simulink model "TotalFramework"  (Simulink 6.6)
settings: Solver=ode45  StartTime=0.0  StopTime=inf  RelTol=1e-3
libraries: xbsIndex_r4 x42, simulink x4, dspsrcs4 x1, simulink_extras x1
settings Model: Creator=student  LastModifiedBy=student

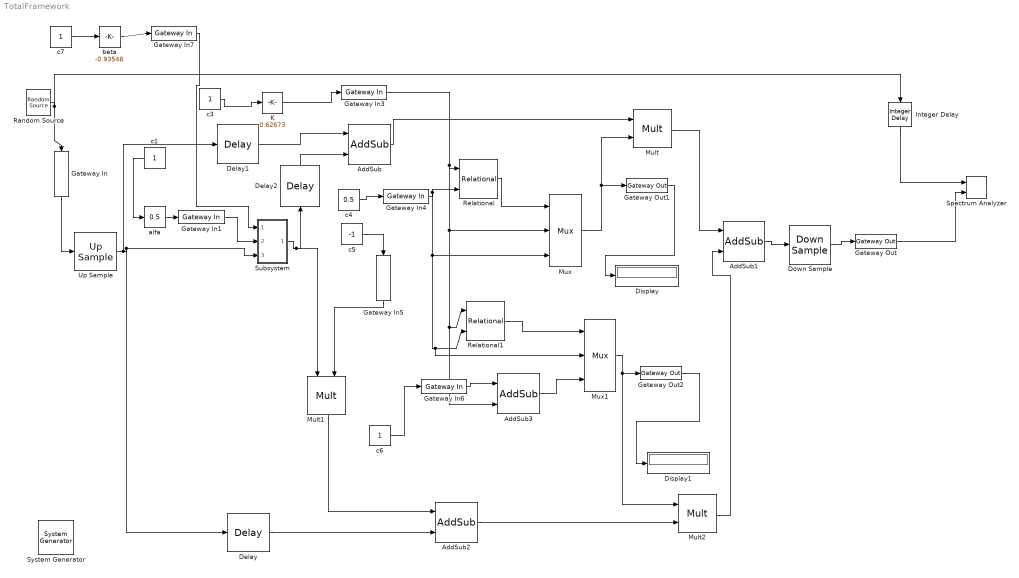
== system TotalFramework ==
  " System Generator" : xbsIndex_r4/ System Generator  Tag=genX  SystemSampleTime=-1  xilinxfamily=virtex4  part=xc4vsx35  speed=-10  package=ff668  synthesis_tool=XST  directory=./netlist  testbench=off  simulink_period=1/10  sysclk_period=10  incr_netlist=off  trim_vbits=Everywhere in SubSystem  dbl_ovrd=According to Block Masks  core_generation=According to Block Masks  run_coregen=off  deprecated_control=off  eval_field=0  block_type=sysgen
      settings: block_version=9.2.00
  AddSub : xbsIndex_r4/AddSub  mode=Addition  use_carryin=off  use_carryout=off  en=off  latency=0  precision=Full  arith_type=Unsigned  n_bits=16  bin_pt=14  quantization=Truncate  overflow=Wrap  dbl_ovrd=off  use_behavioral_HDL=off  pipelined=off  use_rpm=on  block_type=addsub
      settings: block_version=9.2.00
  AddSub1 : xbsIndex_r4/AddSub  mode=Addition  use_carryin=off  use_carryout=off  en=off  latency=2  precision=User Defined  arith_type="Signed  (2's comp)"  n_bits=16  bin_pt=14  quantization=Truncate  overflow=Wrap  dbl_ovrd=off  use_behavioral_HDL=off  pipelined=off  use_rpm=on  block_type=addsub
      settings: block_version=9.2.00
  AddSub2 : xbsIndex_r4/AddSub  mode=Addition  use_carryin=off  use_carryout=off  en=off  latency=0  precision=Full  arith_type=Unsigned  n_bits=16  bin_pt=14  quantization=Truncate  overflow=Wrap  dbl_ovrd=off  use_behavioral_HDL=off  pipelined=off  use_rpm=on  block_type=addsub
      settings: block_version=9.2.00
  AddSub3 : xbsIndex_r4/AddSub  mode=Subtraction  use_carryin=off  use_carryout=off  en=off  latency=0  precision=Full  arith_type=Unsigned  n_bits=16  bin_pt=14  quantization=Truncate  overflow=Wrap  dbl_ovrd=off  use_behavioral_HDL=off  pipelined=off  use_rpm=on  block_type=addsub
      settings: block_version=9.2.00
  Delay : xbsIndex_r4/Delay  en=off  latency=13  dbl_ovrd=off  reg_retiming=off  block_type=delay
      settings: block_version=9.2.00
  Delay1 : xbsIndex_r4/Delay  en=off  latency=13  dbl_ovrd=off  reg_retiming=off  block_type=delay
      settings: block_version=9.2.00
  Delay2 : xbsIndex_r4/Delay  Orientation=up  en=off  latency=3  dbl_ovrd=off  reg_retiming=off  block_type=delay
      settings: block_version=9.2.00
  Display : Display
  Display1 : Display
  Down Sample : xbsIndex_r4/Down Sample  sample_ratio=10  sample_phase=First Value of Frame  en=off  latency=0  dbl_ovrd=off  block_type=dsamp
      settings: block_version=9.2.00
  Gateway In : xbsIndex_r4/Gateway In  Orientation=down  arith_type="Signed  (2's comp)"  n_bits=16  bin_pt=14  quantization="Round  (unbiased: +/- Inf)"  overflow=Saturate  period=1  dbl_ovrd=off  timing_constraint=None  locs_specified=off  LOCs={}  block_type=gatewayin
      settings: infoedit="Gateway in block.  Converts inputs of type Simulink integer, double and fixed point to  Xilinx fixed point type.<P><P>Hardware notes:  In hardware these blocks become top level input ports."  block_version=9.2.00
  Gateway In{1,3..4,6..7} (5 alike) : xbsIndex_r4/Gateway In  arith_type="Signed  (2's comp)"  n_bits=16  bin_pt=14  quantization="Round  (unbiased: +/- Inf)"  overflow=Saturate  period=1  dbl_ovrd=off  timing_constraint=None  locs_specified=off  LOCs={}  block_type=gatewayin
      settings: infoedit="Gateway in block.  Converts inputs of type Simulink integer, double and fixed point to  Xilinx fixed point type.<P><P>Hardware notes:  In hardware these blocks become top level input ports."  block_version=9.2.00
  Gateway In5 : xbsIndex_r4/Gateway In  Orientation=down  arith_type="Signed  (2's comp)"  n_bits=16  bin_pt=14  quantization="Round  (unbiased: +/- Inf)"  overflow=Saturate  period=1  dbl_ovrd=off  timing_constraint=None  locs_specified=off  LOCs={}  block_type=gatewayin
      settings: infoedit="Gateway in block.  Converts inputs of type Simulink integer, double and fixed point to  Xilinx fixed point type.<P><P>Hardware notes:  In hardware these blocks become top level input ports."  block_version=9.2.00
  Gateway Out : xbsIndex_r4/Gateway Out  hdl_port=on  timing_constraint=None  locs_specified=off  LOCs={}  block_type=gatewayout
      settings: infoedit="Gateway out block.  Converts Xilinx fixed point inputs into ouputs of type Simulink integer, double, or fixed point.<P><P>Hardware notes:  In hardware these blocks become top level output ports or are discarded, depending on how they are configured."  block_version=9.2.00
  Gateway Out1 : xbsIndex_r4/Gateway Out  hdl_port=on  timing_constraint=None  locs_specified=off  LOCs={}  block_type=gatewayout
      settings: infoedit="Gateway out block.  Converts Xilinx fixed point inputs into ouputs of type Simulink integer, double, or fixed point.<P><P>Hardware notes:  In hardware these blocks become top level output ports or are discarded, depending on how they are configured."  block_version=9.2.00
  Gateway Out2 : xbsIndex_r4/Gateway Out  hdl_port=on  timing_constraint=None  locs_specified=off  LOCs={}  block_type=gatewayout
      settings: infoedit="Gateway out block.  Converts Xilinx fixed point inputs into ouputs of type Simulink integer, double, or fixed point.<P><P>Hardware notes:  In hardware these blocks become top level output ports or are discarded, depending on how they are configured."  block_version=9.2.00
  Integer Delay : simulink/Discrete/Integer Delay  Orientation=down  vinit=0.0  samptime=1  NumDelays=2
  K : simulink/Math Operations/Slider Gain  SystemSampleTime=-1  low=0  gain=0.62673  high=1
  Mult : xbsIndex_r4/Mult  precision=Full  arith_type="Signed  (2's comp)"  n_bits=16  bin_pt=14  quantization=Truncate  overflow=Wrap  en=off  latency=5  dbl_ovrd=off  use_behavioral_HDL=off  use_embedded=on  opt=Speed  optimum_pipeline=off  pipeline=on  use_rpm=on  placement_style=Triangular  block_type=mult
      settings: infoedit=Hardware notes: To use the internal pipeline stage of the dedicated multiplier you must select 'Pipeline for maximum performance'.  block_version=9.2.00
  Mult1 : xbsIndex_r4/Mult  Orientation=down  precision=Full  arith_type="Signed  (2's comp)"  n_bits=16  bin_pt=14  quantization=Truncate  overflow=Wrap  en=off  latency=3  dbl_ovrd=off  use_behavioral_HDL=off  use_embedded=on  opt=Speed  optimum_pipeline=off  pipeline=on  use_rpm=on  placement_style=Triangular  block_type=mult
      settings: infoedit=Hardware notes: To use the internal pipeline stage of the dedicated multiplier you must select 'Pipeline for maximum performance'.  block_version=9.2.00
  Mult2 : xbsIndex_r4/Mult  precision=Full  arith_type="Signed  (2's comp)"  n_bits=16  bin_pt=14  quantization=Truncate  overflow=Wrap  en=off  latency=5  dbl_ovrd=off  use_behavioral_HDL=off  use_embedded=on  opt=Speed  optimum_pipeline=off  pipeline=on  use_rpm=on  placement_style=Triangular  block_type=mult
      settings: infoedit=Hardware notes: To use the internal pipeline stage of the dedicated multiplier you must select 'Pipeline for maximum performance'.  block_version=9.2.00
  Mux : xbsIndex_r4/Mux  inputs=2  en=off  latency=0  precision=Full  arith_type=Unsigned  n_bits=16  bin_pt=14  quantization=Truncate  overflow=Wrap  dbl_ovrd=off  block_type=mux
      settings: block_version=9.2.00
  Mux1 : xbsIndex_r4/Mux  inputs=2  en=off  latency=0  precision=Full  arith_type=Unsigned  n_bits=16  bin_pt=14  quantization=Truncate  overflow=Wrap  dbl_ovrd=off  block_type=mux
      settings: block_version=9.2.00
  Random Source : dspsrcs4/Random Source  SrcType=Uniform  NormMethod=Ziggurat  CltLength=12  MinVal=-1  MaxVal=+1  MeanVal=0  VarVal=1  RepMode=Not repeatable  rawSeed=1  IsInherit=off  SampMode=Discrete  SampTime=1  SampFrame=1  DataType=Double  OutComplex=Real
  Relational : xbsIndex_r4/Relational  mode=a>b  en=off  latency=1  dbl_ovrd=off  block_type=relational
      settings: block_version=9.2.00
  Relational1 : xbsIndex_r4/Relational  mode=a>b  en=off  latency=1  dbl_ovrd=off  block_type=relational
      settings: block_version=9.2.00
  Spectrum Analyzer : simulink_extras/Additional Sinks/Spectrum Analyzer  SystemSampleTime=-1  npts=1024  fftpts=1024  HowOften=64  sampleT=1
  Subsystem : Subsystem
  Up Sample : xbsIndex_r4/Up Sample  sample_ratio=10  copy_samples=off  dbl_ovrd=off  block_type=usamp
      settings: infoedit="Up samples input data.  Inserted values  can be zeros or copies of the most recent input sample.<P><P>Hardware notes: No hardware is needed if inserted values are copies of the input sample; otherwise, a mux and single bit flip-flop are used."  block_version=9.2.00
  alfa : simulink/Math Operations/Slider Gain  SystemSampleTime=-1  low=0  gain=0.5  high=1
  beta : simulink/Math Operations/Slider Gain  SystemSampleTime=-1  low=-1  gain=-0.93548  high=1
  c1 : Constant  Orientation=left
  c3 : Constant
  c4 : Constant  Value=0.5
  c5 : Constant  Value=-1
  c6 : Constant
  c7 : Constant
  wires:
  Random Source/1 -> Gateway In/1, Integer Delay/1
  c1/1 -> alfa/1
  alfa/1 -> Gateway In1/1
  Gateway Out/1 -> Spectrum Analyzer/2
  Subsystem/1(Out1) -> Mult1/1, Delay2/1
  c3/1 -> K/1
  K/1 -> Gateway In3/1
  c4/1 -> Gateway In4/1
  Gateway In4/1 -> Relational/2, Mux/3, Relational1/2, Mux1/2
  Gateway In3/1 -> Relational/1, Mux/2, Relational1/1, AddSub3/2
  AddSub/1 -> Mult/1
  Mult/1 -> AddSub1/1
  c5/1 -> Gateway In5/1
  Gateway In5/1 -> Mult1/2
  Mult1/1 -> AddSub2/1
  Relational/1 -> Mux/1
  Gateway Out1/1 -> Display/1
  Mux/1 -> Mult/2, Gateway Out1/1
  Relational1/1 -> Mux1/1
  c6/1 -> Gateway In6/1
  Gateway In6/1 -> AddSub3/1
  Gateway Out2/1 -> Display1/1
  Mux1/1 -> Gateway Out2/1, Mult2/1
  Gateway In/1 -> Up Sample/1
  Up Sample/1 -> Delay/1, Subsystem/3(input), Delay1/1
  Down Sample/1 -> Gateway Out/1
  AddSub1/1 -> Down Sample/1
  AddSub2/1 -> Mult2/2
  Mult2/1 -> AddSub1/2
  AddSub3/1 -> Mux1/3
  Integer Delay/1 -> Spectrum Analyzer/1
  Delay/1 -> AddSub2/2
  Delay1/1 -> AddSub/1
  Delay2/1 -> AddSub/2
  Gateway In1/1 -> Subsystem/2(alfa)
  c7/1 -> beta/1
  beta/1 -> Gateway In7/1
  Gateway In7/1 -> Subsystem/1(In1)

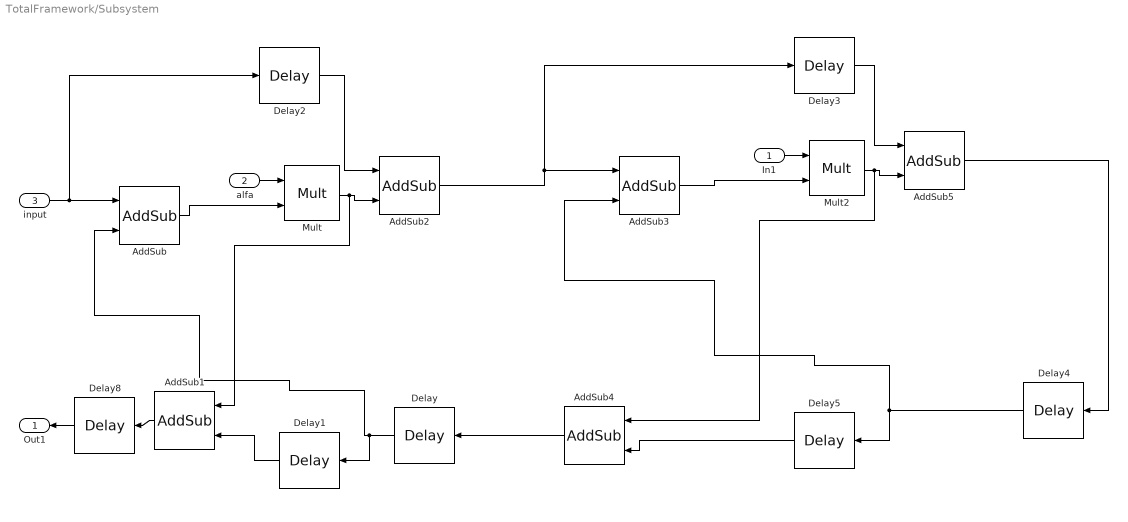
== system TotalFramework/Subsystem ==
  In1 : Inport
  alfa : Inport  Port=2
  input : Inport  Port=3
  AddSub : xbsIndex_r4/AddSub  mode=Subtraction  use_carryin=off  use_carryout=off  en=off  latency=0  precision=Full  arith_type="Signed  (2's comp)"  n_bits=16  bin_pt=14  quantization=Truncate  overflow=Wrap  dbl_ovrd=off  use_behavioral_HDL=off  pipelined=off  use_rpm=on  block_type=addsub
      settings: block_version=9.2.00
  AddSub1 : xbsIndex_r4/AddSub  Orientation=left  mode=Addition  use_carryin=off  use_carryout=off  en=off  latency=0  precision=User Defined  arith_type="Signed  (2's comp)"  n_bits=16  bin_pt=14  quantization=Truncate  overflow=Wrap  dbl_ovrd=off  use_behavioral_HDL=off  pipelined=off  use_rpm=on  block_type=addsub
      settings: block_version=9.2.00
  AddSub2 : xbsIndex_r4/AddSub  mode=Addition  use_carryin=off  use_carryout=off  en=off  latency=0  precision=Full  arith_type=Unsigned  n_bits=16  bin_pt=14  quantization=Truncate  overflow=Wrap  dbl_ovrd=off  use_behavioral_HDL=off  pipelined=off  use_rpm=on  block_type=addsub
      settings: block_version=9.2.00
  AddSub3 : xbsIndex_r4/AddSub  mode=Subtraction  use_carryin=off  use_carryout=off  en=off  latency=0  precision=Full  arith_type="Signed  (2's comp)"  n_bits=16  bin_pt=14  quantization=Truncate  overflow=Wrap  dbl_ovrd=off  use_behavioral_HDL=off  pipelined=off  use_rpm=on  block_type=addsub
      settings: block_version=9.2.00
  AddSub4 : xbsIndex_r4/AddSub  Orientation=left  mode=Addition  use_carryin=off  use_carryout=off  en=off  latency=0  precision=Full  arith_type=Unsigned  n_bits=16  bin_pt=14  quantization=Truncate  overflow=Wrap  dbl_ovrd=off  use_behavioral_HDL=off  pipelined=off  use_rpm=on  block_type=addsub
      settings: block_version=9.2.00
  AddSub5 : xbsIndex_r4/AddSub  mode=Addition  use_carryin=off  use_carryout=off  en=off  latency=0  precision=Full  arith_type=Unsigned  n_bits=16  bin_pt=14  quantization=Truncate  overflow=Wrap  dbl_ovrd=off  use_behavioral_HDL=off  pipelined=off  use_rpm=on  block_type=addsub
      settings: block_version=9.2.00
  Delay : xbsIndex_r4/Delay  Orientation=left  en=off  latency=4  dbl_ovrd=off  reg_retiming=off  block_type=delay
      settings: block_version=9.2.00
  Delay1 : xbsIndex_r4/Delay  Orientation=left  en=off  latency=3  dbl_ovrd=off  reg_retiming=off  block_type=delay
      settings: block_version=9.2.00
  Delay2 : xbsIndex_r4/Delay  en=off  latency=3  dbl_ovrd=off  reg_retiming=off  block_type=delay
      settings: block_version=9.2.00
  Delay3 : xbsIndex_r4/Delay  en=off  latency=3  dbl_ovrd=off  reg_retiming=off  block_type=delay
      settings: block_version=9.2.00
  Delay4 : xbsIndex_r4/Delay  Orientation=left  en=off  latency=7  dbl_ovrd=off  reg_retiming=off  block_type=delay
      settings: block_version=9.2.00
  Delay5 : xbsIndex_r4/Delay  Orientation=left  en=off  latency=3  dbl_ovrd=off  reg_retiming=off  block_type=delay
      settings: block_version=9.2.00
  Delay8 : xbsIndex_r4/Delay  Orientation=left  en=off  latency=7  dbl_ovrd=off  reg_retiming=off  block_type=delay
      settings: block_version=9.2.00
  Mult : xbsIndex_r4/Mult  precision=User Defined  arith_type="Signed  (2's comp)"  n_bits=20  bin_pt=14  quantization=Truncate  overflow=Wrap  en=off  latency=3  dbl_ovrd=off  use_behavioral_HDL=off  use_embedded=on  opt=Speed  optimum_pipeline=off  pipeline=on  use_rpm=on  placement_style=Triangular  block_type=mult
      settings: infoedit=Hardware notes: To use the internal pipeline stage of the dedicated multiplier you must select 'Pipeline for maximum performance'.  block_version=9.2.00
  Mult2 : xbsIndex_r4/Mult  precision=User Defined  arith_type="Signed  (2's comp)"  n_bits=24  bin_pt=14  quantization=Truncate  overflow=Wrap  en=off  latency=3  dbl_ovrd=off  use_behavioral_HDL=off  use_embedded=on  opt=Speed  optimum_pipeline=off  pipeline=on  use_rpm=on  placement_style=Triangular  block_type=mult
      settings: infoedit=Hardware notes: To use the internal pipeline stage of the dedicated multiplier you must select 'Pipeline for maximum performance'.  block_version=9.2.00
  Out1 : Outport  Orientation=left
  wires:
  input/1 -> Delay2/1, AddSub/1
  Delay1/1 -> AddSub1/2
  AddSub1/1 -> Delay8/1
  Delay5/1 -> AddSub4/2
  AddSub5/1 -> Delay4/1
  Delay4/1 -> Delay5/1, AddSub3/2
  Delay3/1 -> AddSub5/1
  Delay2/1 -> AddSub2/1
  AddSub4/1 -> Delay/1
  AddSub2/1 -> AddSub3/1, Delay3/1
  Mult2/1 -> AddSub5/2, AddSub4/1
  AddSub3/1 -> Mult2/2
  Delay/1 -> AddSub/2, Delay1/1
  Mult/1 -> AddSub2/2, AddSub1/1
  AddSub/1 -> Mult/2
  In1/1 -> Mult2/1
  alfa/1 -> Mult/1
  Delay8/1 -> Out1/1
